simulink model "dcmotorspeedcontrol"  (R2013a)
settings: Solver=ode3  StartTime=1.0  StopTime=2.0  FixedStep=Ts  RelTol=1e-3
values from neighbouring files (symbols this model uses):
  A = ones(5 ,7)    [Exp_1.m]    (also in Q7.m = [1 1 0 1 0 ; 0 -1 1 0 1 ])
  Raext = 1e-20    [dcmotor.m]
  Rfext = 1e-20    [dcmotor.m]
  TL = Torque(i)    [dcmotor.m]
  Torque = 0:50:500    [dcmotor.m]
  Ts = 0.01    [dcmotor.m]
  Vf = 240    [dcmotor.m]
  Vt = .026    (= 0.026)    [Exp_1_part2a.m]    (also in dcmotor.m = Va(j))
libraries: powerlib x10, simeventslib x2
settings Model: Creator=Saran Satsangi  LastModifiedBy=Saran Satsangi

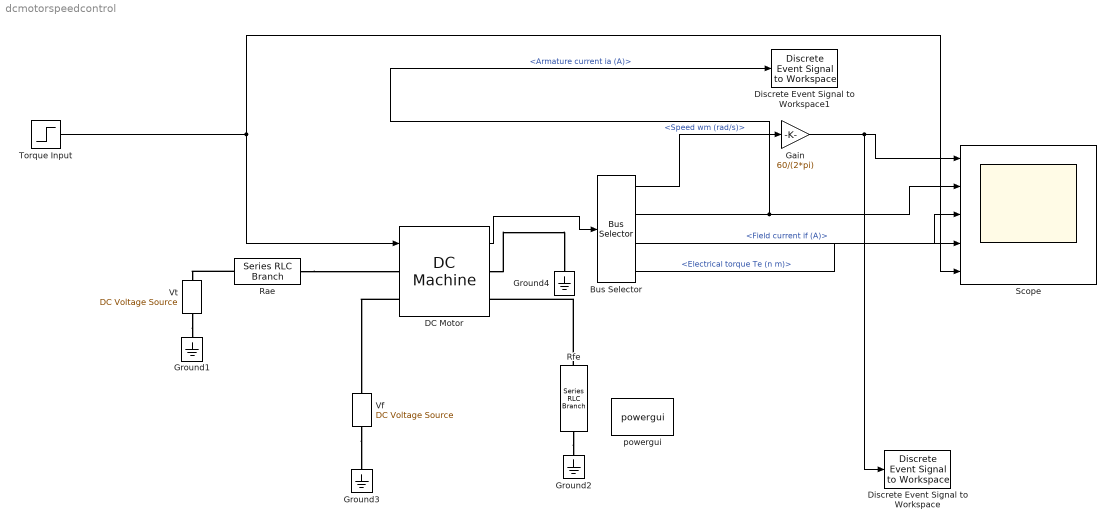
== system dcmotorspeedcontrol ==
  Bus Selector : BusSelector  OutputSignals=Speed wm (rad/s),Armature current ia (A),Field current if (A),Electrical torque Te (n m)
  DC Motor : powerlib/Machines/DC Machine  PresetModel=No  MechanicalLoad=Torque TL  FieldType=Wound  ShowDetailedParameters=on  RLa=[ 0.6 0.012]  RLf="[ 240  120]"  Laf=1.8  MachineConstant=Torque constant (N.m/A)  Ke=1.8  Kt=1.8  J=1  Bm=0  Tf=0  w0=1  Ifinit=1  TsPowergui=0  TsBlock=-1
  Discrete Event Signal to Workspace : simeventslib/SimEvents Sinks/Discrete Event Signal to Workspace  VariableName=Y  SaveFormat=Array  isMonitorOnly=off  isRecordIC=off
  Discrete Event Signal to Workspace1 : simeventslib/SimEvents Sinks/Discrete Event Signal to Workspace  VariableName=X  SaveFormat=Array  isMonitorOnly=off  isRecordIC=off
  Gain : Gain  Gain=60/(2*pi)
  Ground{1..4} (4 alike) : powerlib/Elements/Ground  LConnTagsString=a
  Rae : powerlib/Elements/Series RLC Branch  LConnTagsString=__new0  RConnTagsString=__new0  BranchType=R  Resistance=Raext  Inductance=1e-3  SetiL0=off  InitialCurrent=0  Capacitance=1e-6  Setx0=off  InitialVoltage=0  Measurements=None
  Rfe : powerlib/Elements/Series RLC Branch  LConnTagsString=__new0  RConnTagsString=__new0  BranchType=R  Resistance=Rfext  Inductance=1e-3  SetiL0=off  InitialCurrent=0  Capacitance=1e-6  Setx0=off  InitialVoltage=0  Measurements=None
  Scope : Scope  NumInputPorts=5
      settings: YMin=-5~-5~-5~-5~-5  YMax=5~5~5~5~5
  Torque Input : Step  After=TL  SampleTime=Ts
  Vf : powerlib/Electrical Sources/DC Voltage Source  Amplitude=Vf  Measurements=None
  Vt : powerlib/Electrical Sources/DC Voltage Source  Amplitude=Vt  Measurements=None
  powergui : powerlib/powergui  Priority=1  SimulationMode=Discrete  SolverType=Tustin  SampleTime=Ts  frequency=60  SPID=off  DisableSnubberDevices=off  DisableRonSwitches=off  DisableVfSwitches=off  SwTol=0  Interpol=off  DisplayEquations=off  frequencyindice=0  Pbase=100e6  ErrMax=1e-4  Iterations=50  UnitsV=kV  UnitsW=MW  FunctionMessages=off  echomessages=off  HookPort=off  EnableUseOfTLC=off  x0status=blocks  RestoreLinks=warning  ResistiveCurrentMeasurement=off  Frange=[0:2:500]  Ylog=off  Xlog=on  ShowGrid=off  save=off  variable=ZData  ZoomFFT=off  StartTime=0.0  cycles=1  DisplayStyle=1  fundamental=60  FreqAxis=off  MaxFrequency=1000  frequencyindicesteady=1  RmsSteady=1  display=off  Ts=0  methode=off
  wires:
  Bus Selector/1 -> Gain/1  "<Speed wm (rad/s)>"
  Bus Selector/2 -> Discrete Event Signal to Workspace1/1, Scope/2  "<Armature current ia (A)>"
  Bus Selector/3 -> Scope/3  "<Field current if (A)>"
  Bus Selector/4 -> Scope/4  "<Electrical torque Te (n m)>"
  Torque Input/1 -> DC Motor/1, Scope/5
  DC Motor/1 -> Bus Selector/1
  Gain/1 -> Discrete Event Signal to Workspace/1, Scope/1
  connections:
  Vt/LConn1 -- Ground1/LConn1
  DC Motor/LConn2 -- Vf/RConn1
  DC Motor/RConn1 -- Ground4/LConn1
  Rfe/LConn1 -- DC Motor/RConn2
  Rfe/RConn1 -- Ground2/LConn1
  Vf/LConn1 -- Ground3/LConn1
  Rae/RConn1 -- DC Motor/LConn1
  Rae/LConn1 -- Vt/RConn1
